simulink model "A7_S42"  (R2015a)
settings: Solver=ode45  StartTime=20  StopTime=1000  RelTol=1e-3
settings Model: Creator=James  LastModifiedBy=James

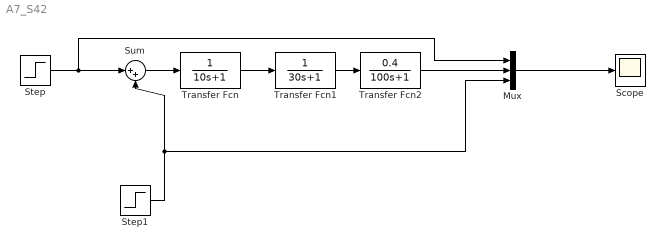
== system A7_S42 ==
  Mux : Mux  Inputs=3
  Scope : Scope
      settings: YMax=15
  Step : Step  Time=0  After=50  SampleTime=0
  Step1 : Step  Time=400  After=20  SampleTime=0
  Sum : Sum  Inputs=|++
  Transfer Fcn : TransferFcn  Denominator=[10 1]
  Transfer Fcn1 : TransferFcn  Denominator=[30 1]
  Transfer Fcn2 : TransferFcn  Numerator=[0.4]  Denominator=[100 1]
  wires:
  Step/1 -> Mux/1, Sum/1
  Sum/1 -> Transfer Fcn/1
  Mux/1 -> Scope/1
  Transfer Fcn/1 -> Transfer Fcn1/1
  Transfer Fcn1/1 -> Transfer Fcn2/1
  Transfer Fcn2/1 -> Mux/2
  Step1/1 -> Mux/3, Sum/2
